simulink model "sampleModel1788"  (R2023a)
settings: Solver=VariableStepAuto  StartTime=0.0  StopTime=10.0  RelTol=1e-3
libraries: hdlsllib x8, simulink x3
settings Model: Creator=user1  LastModifiedBy=user1

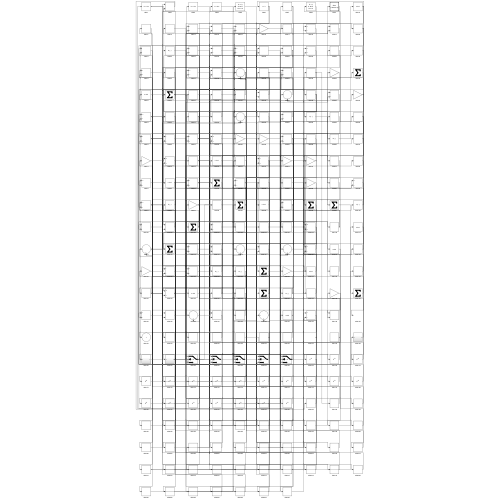
[thumbnail: Simulink's stored preview of the top-level diagram]
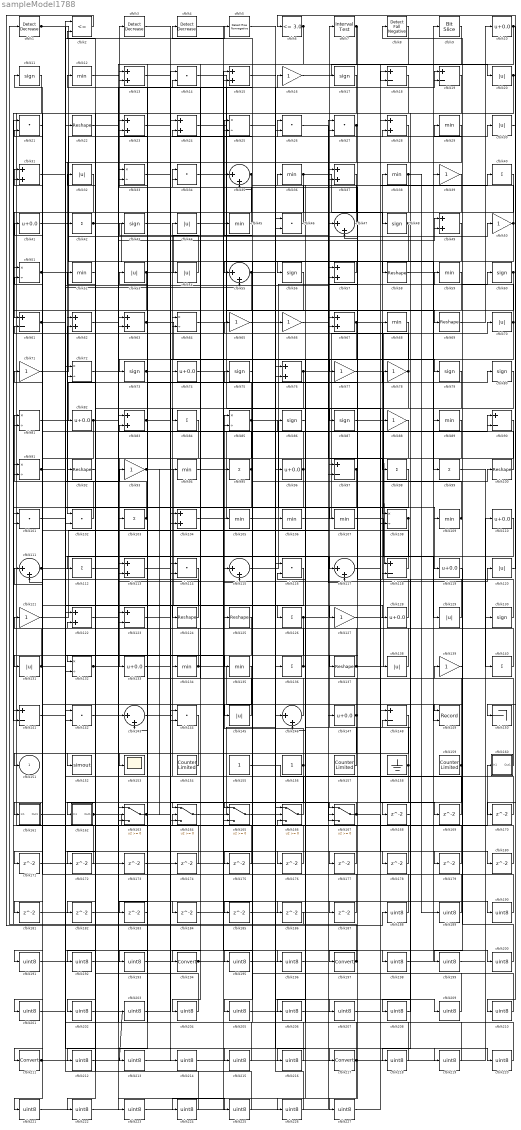
== system sampleModel1788 ==
  cfblk1 : simulink/Logic and Bit Operations/Detect Decrease  vinit=0.0  OutDataTypeStr=boolean
      settings: LibrarySourceBlock=|
      | hdlsllib/Logic and Bit
      | Operations/Detect
      | Decrease
  cfblk{10,41,74,82,96,110,119,128,133,147} (10 alike) : Bias  Bias=0.0  SaturateOnIntegerOverflow=off
  cfblk{22,58,69,92,100,124..125,137} (8 alike) : Reshape
  cfblk{14,21,26..27,34,46,101..102,114,116,142,144} (12 alike) : DotProduct  OutDataTypeStr=Inherit: Inherit via internal rule
  cfblk{40,42,84,95,98..99,103,112,126,136,140} (11 alike) : Sum  Inputs=+
  cfblk{13,15,23..24,28,31,37,49,57,62..63,67,76,83,104,113,122} (17 alike) : Sum
  cfblk{12,29,36,38,45,52,59,68,89,94,105..107,109,134..135} (16 alike) : MinMax
  cfblk{25,33,51,64,72,81,85,91,108,132} (10 alike) : Product  Inputs=*/  RndMeth=Zero  SaturateOnIntegerOverflow=on
  cfblk{11,17,43,48,56,60,73,75,79..80,86..87,130} (13 alike) : Signum
  cfblk{35,47,55,111,115,117,143,146} (8 alike) : Sum  Inputs=|++
  cfblk{18..19,61,90,97,118,123,141,148} (9 alike) : Sum  Inputs=+-
  cfblk{20,30,32,44,53..54,70,120,129,131,138,145} (12 alike) : Abs  SaturateOnIntegerOverflow=off
  cfblk{16,39,50,65..66,71,77..78,88,93,121,127,139} (13 alike) : Gain
  cfblk149 : Record  FileSettingsInternal="{\"entries\":[{\"content\":{\"excelSettings\":{\"content\":{},\"type\":\"Streamout.ExcelSettings\"}},\"type\":\"Streamout.FileSettingStorage\",\"uuid\":\"\"}],\"packageUris\":[\"http:\\/\\/schema.mathworks.com\\/mf0\\/streamout_blocks\\/R2020a\"],\"version\":\"1.0\"}"  Layout=[1 1]  SignalsInternal="{\"entries\":[{\"content\":{\"signals\":[{\"content\":{\"blockPath\":[],\"dimensions\":[1],\"domain\":\"\",\"lineColor\":\"#a2142f\",\"plots\":[1],\"port\":1,\"signalID\":4068,\"signalName\":\"XY Graph:1\"},\"type\":\"RecordBlkView.Signal\",\"uuid\":\"\"},{\"content\":{\"blockPath\":[],\"dimensions\":[1],\"domain\":\"\",\"lineColor\":\"#139fff\",\"plots\":[1],\"port\":2,\"signalID\":4071,\"signalName\":\"XY Graph:2\"},\"type\":\"RecordBlkView.Signal\",\"uuid\":\"\"}]},\"type\":\"RecordBlkView.InputSignals\",\"uuid\":\"\"}],\"packageUris\":[\"http:\\/\\/schema.mathworks.com\\/mf0\\/streamout_blocks\\/R2020a\"],\"version\":\"1.0\"}"  VisualizationBindings="{\"xyplotplugin\":{\"info\":[{\"series\":[{\"bindingParametersList\":[{\"parameter\":\"X-Axis\",\"signalID\":4068,\"signalName\":\"XY Graph:1\"},{\"parameter\":\"Y-Axis\",\"signalID\":4071,\"signalName\":\"XY Graph:2\"}],\"seriesID\":38091}],\"subplotID\":1}]}}"  CompatibilityTag=XY  st=-1
  cfblk150 : Terminator
  cfblk152 : ToWorkspace  VariableName=simout  SaveFormat=Timeseries  SampleTime=-1
  cfblk153 : Scope
  cfblk154 : hdlsllib/Sources/Counter Limited  uplimit=7  tsamp=-1
  cfblk155 : Constant  SampleTime=-1
  cfblk156 : Constant  SampleTime=-1
  cfblk157 : hdlsllib/Sources/Counter Limited  uplimit=7  tsamp=-1
  cfblk158 : Ground
  cfblk159 : hdlsllib/Sources/Counter Limited  uplimit=7  tsamp=-1
  cfblk160 : Subsystem
      settings: LibrarySourceBlock=|
      | hdlsllib/Ports &
      | Subsystems/Subsystem
  cfblk161 : Subsystem
      settings: LibrarySourceBlock=|
      | hdlsllib/Ports &
      | Subsystems/Subsystem
  cfblk162 : Subsystem
      settings: LibrarySourceBlock=|
      | hdlsllib/Ports &
      | Subsystems/Subsystem
  cfblk{163..167} (5 alike) : Switch  SaturateOnIntegerOverflow=off  InputSameDT=off
  cfblk{168..187} (20 alike) : Delay  SampleTime=1
  cfblk{188..193,195..196,198..210,212..216,218..227} (36 alike) : DataTypeConversion  OutDataTypeStr=uint8  SaturateOnIntegerOverflow=off  RndMeth=Floor
  cfblk{194,197,211,217} (4 alike) : DataTypeConversion  SaturateOnIntegerOverflow=off  RndMeth=Floor
  cfblk2 : RelationalOperator  Operator=<=  OutDataTypeStr=boolean  InputSameDT=off
  cfblk3 : simulink/Logic and Bit Operations/Detect Decrease  vinit=0.0  OutDataTypeStr=boolean
      settings: LibrarySourceBlock=|
      | hdlsllib/Logic and Bit
      | Operations/Detect
      | Decrease
  cfblk4 : simulink/Logic and Bit Operations/Detect Decrease  vinit=0.0  OutDataTypeStr=boolean
      settings: LibrarySourceBlock=|
      | hdlsllib/Logic and Bit
      | Operations/Detect
      | Decrease
  cfblk5 : hdlsllib/Logic and Bit Operations/Detect Rise Nonnegative  vinit=0  OutDataTypeStr=boolean
  cfblk6 : hdlsllib/Logic and Bit Operations/Compare To Constant  relop=<=  const=3.0  OutDataTypeStr=boolean
  cfblk7 : hdlsllib/Logic and Bit Operations/Interval Test  IntervalClosedRight=on  uplimit=0.5  IntervalClosedLeft=on  lowlimit=-0.5  OutDataTypeStr=boolean
  cfblk8 : hdlsllib/Logic and Bit Operations/Detect Fall Negative  vinit=0  OutDataTypeStr=boolean
  cfblk9 : hdlsllib/Logic and Bit Operations/Bit Slice  lidx=7  ridx=0
  cfblk151 : Outport  VectorParamsAs1DForOutWhenUnconnected=off
  wires:
  cfblk115/1 -> cfblk59/1
  cfblk45/1 -> cfblk3/1
  cfblk156/1 -> cfblk85/1, cfblk163/3
  cfblk155/1 -> cfblk8/1
  cfblk71/1 -> cfblk30/1
  cfblk128/1 -> cfblk38/1
  cfblk86/1 -> cfblk146/2
  cfblk158/1 -> cfblk7/1, cfblk213/1
  cfblk137/1 -> cfblk100/1, cfblk83/2, cfblk132/1
  cfblk38/1 -> cfblk73/1, cfblk189/1
  cfblk165/1 -> cfblk106/1
  cfblk120/1 -> cfblk6/1
  cfblk11/1 -> cfblk160/1(In1)
  cfblk102/1 -> cfblk81/1
  cfblk32/1 -> cfblk102/1
  cfblk134/1 -> cfblk71/1, cfblk149/2, cfblk51/2
  cfblk70/1 -> cfblk29/1, cfblk113/2, cfblk208/1
  cfblk10/1 -> cfblk18/2, cfblk170/1
  cfblk17/1 -> cfblk81/2
  cfblk157/1 -> cfblk34/1
  cfblk104/1 -> cfblk28/1
  cfblk166/1 -> cfblk44/1
  cfblk127/1 -> cfblk70/1
  cfblk35/1 -> cfblk61/1, cfblk42/1
  cfblk27/1 -> cfblk62/1, cfblk132/2
  cfblk106/1 -> cfblk39/1
  cfblk67/1 -> cfblk118/1, cfblk124/1
  cfblk95/1 -> cfblk101/2, cfblk64/2
  cfblk64/1 -> cfblk26/1
  cfblk126/1 -> cfblk142/2, cfblk90/1
  cfblk90/1 -> cfblk145/1
  cfblk51/1 -> cfblk50/1, cfblk108/1
  cfblk164/1 -> cfblk46/1
  cfblk124/1 -> cfblk31/1
  cfblk36/1 -> cfblk48/1, cfblk123/2
  cfblk56/1 -> cfblk153/1
  cfblk154/1 -> cfblk151/1
  cfblk84/1 -> cfblk133/1
  cfblk14/1 -> cfblk138/1
  cfblk1/1 -> cfblk56/1, cfblk219/1
  cfblk58/1 -> cfblk89/1
  cfblk121/1 -> cfblk66/1
  cfblk81/1 -> cfblk80/1
  cfblk119/1 -> cfblk149/1
  cfblk93/1 -> cfblk127/1, cfblk183/1
  cfblk141/1 -> cfblk5/1
  cfblk132/1 -> cfblk163/1, cfblk19/2
  cfblk103/1 -> cfblk62/2, cfblk13/2
  cfblk8/1 -> cfblk46/2
  cfblk46/1 -> cfblk4/1
  cfblk147/1 -> cfblk14/2, cfblk152/1
  cfblk7/1 -> cfblk84/1, cfblk117/1
  cfblk146/1 -> cfblk23/1
  cfblk97/1 -> cfblk57/1, cfblk216/1
  cfblk78/1 -> cfblk11/1, cfblk108/2
  cfblk161/1(Out1) -> cfblk22/1
  cfblk16/1 -> cfblk20/1
  cfblk9/1 -> cfblk197/1
  cfblk145/1 -> cfblk53/1
  cfblk54/1 -> cfblk13/1
  cfblk92/1 -> cfblk32/1
  cfblk112/1 -> cfblk143/1
  cfblk85/1 -> cfblk119/1, cfblk43/1, cfblk212/1
  cfblk136/1 -> cfblk64/1, cfblk36/1
  cfblk110/1 -> cfblk162/1(In1)
  cfblk130/1 -> cfblk34/2
  cfblk131/1 -> cfblk121/1, cfblk163/2, cfblk135/1, cfblk180/1
  cfblk29/1 -> cfblk143/2
  cfblk39/1 -> cfblk113/1
  cfblk61/1 -> cfblk82/1, cfblk57/2, cfblk117/2
  cfblk72/1 -> cfblk217/1
  cfblk99/1 -> cfblk140/1
  cfblk66/1 -> cfblk60/1
  cfblk100/1 -> cfblk52/1
  cfblk111/1 -> cfblk97/1, cfblk55/2
  cfblk4/1 -> cfblk105/1
  cfblk162/1(Out1) -> cfblk75/1, cfblk49/2, cfblk164/2
  cfblk43/1 -> cfblk77/1
  cfblk12/1 -> cfblk123/1
  cfblk142/1 -> cfblk120/1
  cfblk63/1 -> cfblk28/2, cfblk96/1, cfblk167/3
  cfblk143/1 -> cfblk134/1
  cfblk30/1 -> cfblk150/1
  cfblk77/1 -> cfblk109/1
  cfblk24/1 -> cfblk69/1
  cfblk3/1 -> cfblk76/2
  cfblk69/1 -> cfblk10/1
  cfblk91/1 -> cfblk128/1, cfblk196/1
  cfblk34/1 -> cfblk16/1
  cfblk55/1 -> cfblk141/2, cfblk17/1
  cfblk44/1 -> cfblk25/1
  cfblk82/1 -> cfblk19/1, cfblk111/2, cfblk90/2
  cfblk113/1 -> cfblk49/1
  cfblk49/1 -> cfblk107/1
  cfblk31/1 -> cfblk126/1
  cfblk117/1 -> cfblk40/1
  cfblk6/1 -> cfblk63/2, cfblk193/1
  cfblk57/1 -> cfblk55/1
  cfblk138/1 -> cfblk85/2
  cfblk47/1 -> cfblk12/1
  cfblk80/1 -> cfblk87/1
  cfblk76/1 -> cfblk79/1, cfblk165/1, cfblk112/1, cfblk205/1
  cfblk167/1 -> cfblk164/1, cfblk179/1
  cfblk83/1 -> cfblk166/2, cfblk215/1
  cfblk160/1(Out1) -> cfblk86/1
  cfblk60/1 -> cfblk103/1, cfblk167/1
  cfblk123/1 -> cfblk24/1
  cfblk73/1 -> cfblk167/2, cfblk186/1
  cfblk26/1 -> cfblk98/1
  cfblk159/1 -> cfblk45/1, cfblk164/3
  cfblk53/1 -> cfblk47/1, cfblk161/1(In1)
  cfblk116/1 -> cfblk194/1
  cfblk42/1 -> cfblk99/1, cfblk187/1
  cfblk163/1 -> cfblk54/1, cfblk94/1, cfblk178/1
  cfblk129/1 -> cfblk74/1
  cfblk41/1 -> cfblk115/1
  cfblk20/1 -> cfblk131/1, cfblk210/1
  cfblk107/1 -> cfblk129/1
  cfblk140/1 -> cfblk91/1
  cfblk101/1 -> cfblk93/1
  cfblk48/1 -> cfblk78/1, cfblk165/2, cfblk185/1
  cfblk96/1 -> cfblk21/2, cfblk192/1
  cfblk108/1 -> cfblk165/3, cfblk182/1
  cfblk5/1 -> cfblk136/1
  cfblk40/1 -> cfblk91/2
  cfblk50/1 -> cfblk24/2, cfblk137/1
  cfblk98/1 -> cfblk104/2
  cfblk109/1 -> cfblk35/1, cfblk47/2
  cfblk19/1 -> cfblk58/1
  cfblk37/1 -> cfblk211/1
  cfblk118/1 -> cfblk31/2
  cfblk89/1 -> cfblk168/1
  cfblk87/1 -> cfblk169/1
  cfblk169/1 -> cfblk104/1
  cfblk170/1 -> cfblk142/1
  cfblk125/1 -> cfblk171/1
  cfblk171/1 -> cfblk14/1
  cfblk52/1 -> cfblk172/1
  cfblk172/1 -> cfblk111/1
  cfblk62/1 -> cfblk173/1
  cfblk173/1 -> cfblk146/1
  cfblk13/1 -> cfblk174/1
  cfblk174/1 -> cfblk83/1
  cfblk75/1 -> cfblk175/1
  cfblk175/1 -> cfblk101/1
  cfblk74/1 -> cfblk176/1
  cfblk176/1 -> cfblk141/1
  cfblk105/1 -> cfblk177/1
  cfblk177/1 -> cfblk61/2
  cfblk178/1 -> cfblk25/2
  cfblk179/1 -> cfblk118/2
  cfblk180/1 -> cfblk51/1
  cfblk135/1 -> cfblk181/1
  cfblk181/1 -> cfblk63/1
  cfblk183/1 -> cfblk23/2
  cfblk22/1 -> cfblk184/1
  cfblk184/1 -> cfblk67/1
  cfblk185/1 -> cfblk97/2
  cfblk186/1 -> cfblk1/1
  cfblk187/1 -> cfblk35/2
  cfblk2/1 -> cfblk188/1
  cfblk188/1 -> cfblk41/1
  cfblk189/1 -> cfblk2/1
  cfblk133/1 -> cfblk190/1
  cfblk190/1 -> cfblk2/2
  cfblk144/1 -> cfblk191/1
  cfblk191/1 -> cfblk95/1
  cfblk192/1 -> cfblk144/1
  cfblk193/1 -> cfblk144/2
  cfblk194/1 -> cfblk26/2, cfblk67/2
  cfblk79/1 -> cfblk195/1
  cfblk195/1 -> cfblk116/1
  cfblk196/1 -> cfblk116/2
  cfblk197/1 -> cfblk21/1, cfblk76/1
  cfblk23/1 -> cfblk198/1
  cfblk198/1 -> cfblk9/1
  cfblk139/1 -> cfblk199/1
  cfblk199/1 -> cfblk110/1
  cfblk94/1 -> cfblk200/1
  cfblk200/1 -> cfblk139/1
  cfblk114/1 -> cfblk201/1
  cfblk201/1 -> cfblk102/2
  cfblk28/1 -> cfblk202/1
  cfblk202/1 -> cfblk114/1
  cfblk203/1 -> cfblk114/2
  cfblk88/1 -> cfblk204/1
  cfblk204/1 -> cfblk92/1
  cfblk205/1 -> cfblk88/1
  cfblk148/1 -> cfblk206/1
  cfblk206/1 -> cfblk27/2
  cfblk25/1 -> cfblk207/1
  cfblk207/1 -> cfblk148/1
  cfblk208/1 -> cfblk148/2
  cfblk65/1 -> cfblk209/1
  cfblk209/1 -> cfblk27/1
  cfblk210/1 -> cfblk65/1
  cfblk211/1 -> cfblk203/1, cfblk115/2
  cfblk212/1 -> cfblk37/1
  cfblk213/1 -> cfblk37/2
  cfblk33/1 -> cfblk214/1
  cfblk214/1 -> cfblk130/1
  cfblk215/1 -> cfblk33/1
  cfblk216/1 -> cfblk33/2
  cfblk217/1 -> cfblk18/1, cfblk166/3, cfblk224/1
  cfblk168/1 -> cfblk218/1
  cfblk218/1 -> cfblk72/1
  cfblk219/1 -> cfblk72/2
  cfblk15/1 -> cfblk220/1
  cfblk220/1 -> cfblk125/1
  cfblk21/1 -> cfblk221/1
  cfblk221/1 -> cfblk15/1
  cfblk18/1 -> cfblk222/1
  cfblk222/1 -> cfblk15/2
  cfblk122/1 -> cfblk223/1
  cfblk223/1 -> cfblk147/1
  cfblk224/1 -> cfblk122/1
  cfblk182/1 -> cfblk225/1
  cfblk225/1 -> cfblk122/2
  cfblk68/1 -> cfblk226/1
  cfblk226/1 -> cfblk166/1
  cfblk59/1 -> cfblk227/1
  cfblk227/1 -> cfblk68/1

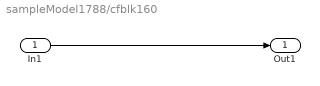
== system sampleModel1788/cfblk160 ==
  In1 : Inport
  Out1 : Outport
  wires:
  In1/1 -> Out1/1

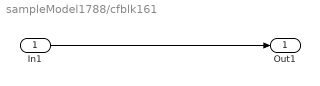
== system sampleModel1788/cfblk161 ==
  In1 : Inport
  Out1 : Outport
  wires:
  In1/1 -> Out1/1

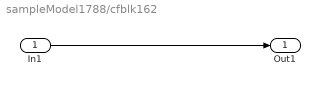
== system sampleModel1788/cfblk162 ==
  In1 : Inport
  Out1 : Outport
  wires:
  In1/1 -> Out1/1
